simulink model "WDS"  (R2022a)
settings: Solver=FixedStepDiscrete  StartTime=0.0  StopTime=T_final  FixedStep=T_sample  RelTol=1e-3
values from neighbouring files (symbols this model uses):
  A_bar_d = readmatrix('A_bar_d.csv')    [Run_model_WDS.m]
  B_bar_d = readmatrix('B_bar_d.csv')    [Run_model_WDS.m]
  BDD_thresh = 5    [Run_model_WDS.m]    (also in run_model.m = 0.05)
  C_obsv_d = readmatrix('C_obsv_d.csv')    [Run_model_WDS.m]    (also in run_model.m = C_obsv; run_model_power_system.m = C_obsv)
  Cm = ones(1,n_states)    [Run_model_WDS.m]
  D_obsv_d = readmatrix('D_obsv_d.csv')    [Run_model_WDS.m]    (also in run_model.m = D_obsv; run_model_power_system.m = D_obsv)
  eta = 0.7    [Run_model_WDS.m]
  H0_perp_full = eye(size(H0_full,1)) - H0_full*H0_full_pinv    [Run_model_WDS.m]    (also in run_model_power_system.m)
  K = place(A_bar_d,B_bar_d,Pc)    [Run_model_WDS.m]
  k0 = 42    [Run_model_WDS.m]
  Lu = F-A_bar_d.'*H0_full_pinv*H1_full    [Run_model_WDS.m]    (also in run_model_power_system.m)
  Ly = A_bar_d.'*H0_full_pinv    [Run_model_WDS.m]    (also in run_model_power_system.m)
  max_attack = 1000    [Run_model_WDS.m]
  n_attack = round(attack_percentage*n_meas)    [Run_model_WDS.m]    (also in run_model.m = round(0.2*n_meas))
  n_meas = size(C_obsv_d,1)    [Run_model_WDS.m]    (also in run_model.m = n_gen + n_bus; run_model_power_system.m = n_gen + n_bus)
  offset = -inv(B_bar_d)*(A_bar_d-eye(n_states))*xd    [Run_model_WDS.m]
  P = [0.69950062422 0.693508114856 0.716853932584 0.638077403246 0.655805243446 0.637952559301 0.64506866417 0.648938826467 0.678776529338 0.684394506866 0.732584269663 0.692634207241 ... (61 elements, 1x61)]    [P.mat]    (also in Run_model_WDS.m = load('P.mat').P.'; detector_evaluation.m = sum(q==q_hat,1)/(size(q,1)); run_model.m = .1 + .4*rand(2*n_gen,1); run_model_power_system.m = .1 + .4*rand(2*n_gen,1))
  Q0 = ones(n_meas,T)    [Run_model_WDS.m]
  r_tau = chi2inv(0.1,n_meas)    [Run_model_WDS.m]
  Sigma = diag(sigma)    [Run_model_WDS.m]    (also in run_model.m)
  sigma_inv_k = 1e2*(3 + 2*rand(n_meas,1))    [Run_model_WDS.m]    (also in run_model.m = 1e4*(3 + 2*rand(m,1)); sigma_inv_k.mat = [541957.05841 17086.3156535 20847.4062112 958.936090052 8825)
  T = round(2*n_states)    [Run_model_WDS.m]    (also in run_model.m = round(2*n); run_model_power_system.m = 10)
  T_sample = 0.01    [Run_model_WDS.m]    (also in run_model.m; run_model_power_system.m)
  T_start_attack = 0.1*T_final    (= 0.8)    [Run_model_WDS.m]    (also in run_model.m = 1.6; run_model_power_system.m)
  T_start_detect = T_start_attack+T*T_sample    [Run_model_WDS.m]    (also in run_model_power_system.m = 0.9)
  U0 = zeros(n_int,T+1)    [Run_model_WDS.m]    (also in run_model.m = zeros(m,T); run_model_power_system.m)
  x0 = zeros(n_states,1)    [Run_model_WDS.m]    (also in run_model.m; run_model_power_system.m)
  xd = 5*ones(n_states,1)    [Run_model_WDS.m]
  Y0 = zeros(n_meas,T)    [Run_model_WDS.m]    (also in run_model.m = zeros(m,T); run_model_power_system.m)
undefined symbols (not defined in the file or in its folder): F, H0_full, H1_full, T_start_opt
libraries: simulink x10
settings Model: Creator=Abelb  LastModifiedBy=Abelb

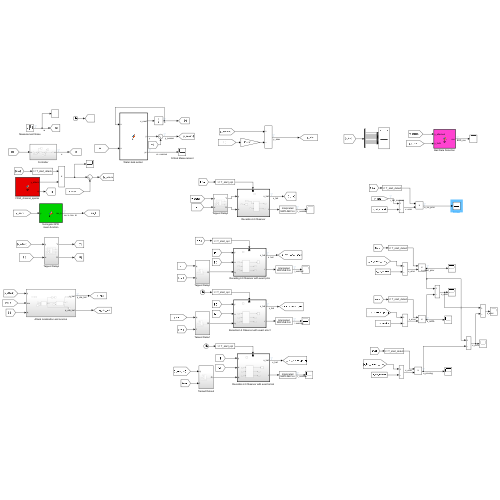
[thumbnail: Simulink's stored preview of the top-level diagram]
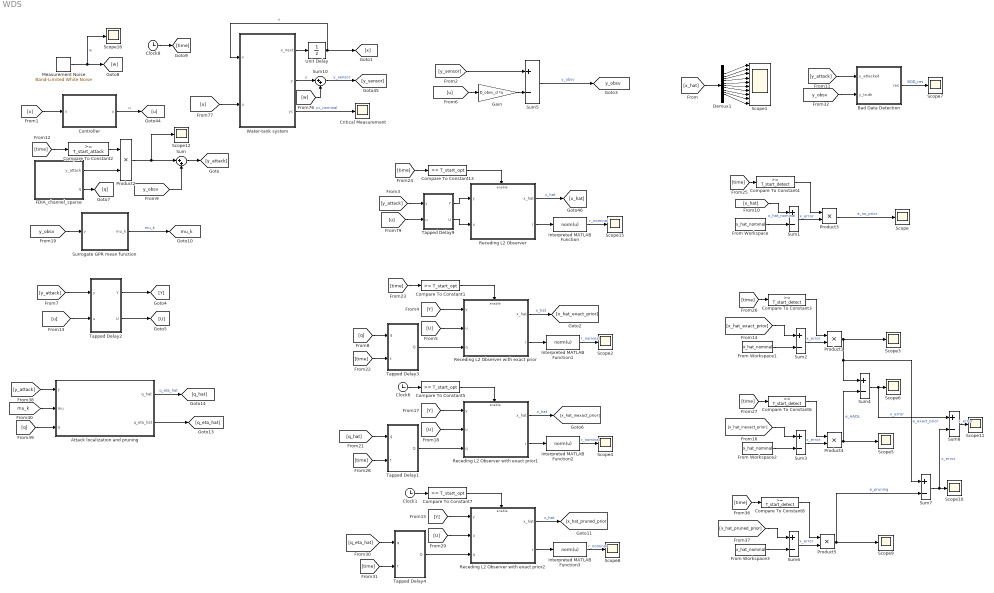
== system WDS ==
  Attack localization and pruning : Subsystem
  Bad Data Detection : MATLAB Function  TreatAsAtomicUnit=on
  Clock1 : Clock
  Clock6 : Clock
  Clock8 : Clock
  Compare To Constant{1,5,7,13} (4 alike) : simulink/Logic and Bit Operations/Compare To Constant  relop=>=  const=T_start_opt  OutDataTypeStr=boolean
  Compare To Constant2 : simulink/Logic and Bit Operations/Compare To Constant  relop=>=  const=T_start_attack  OutDataTypeStr=boolean
  Compare To Constant{3..4,6,8} (4 alike) : simulink/Logic and Bit Operations/Compare To Constant  relop=>=  const=T_start_detect  OutDataTypeStr=boolean
  Controller : Subsystem
  Critical Measurement : Scope
  Demux1 : Demux  Outputs=n_states
  FDIA_channel_sparse : MATLAB Function  TreatAsAtomicUnit=on
  From Workspace{,1..3} (4 alike) : FromWorkspace  VariableName=x_hat_nominal
  Gain : Gain  Gain=D_obsv_d  Multiplication=Matrix(K*u) (u vector)
  Interpreted MATLAB Function{,1..3} (4 alike) : MATLABFcn  MATLABFcn=norm(u)
  Measurement Noise : simulink/Sources/Band-Limited White Noise  Cov=[1e-7]  Ts=T_sample  seed=[23341]
  Product{1..5} (5 alike) : Product
  Receding L2 Observer : Subsystem
  Receding L2 Observer with exact prior : Subsystem
  Receding L2 Observer with exact prior1 : Subsystem
  Receding L2 Observer with exact prior2 : Subsystem
  Scope{,2..12,15..16} (14 alike) : Scope
  Scope1 : Scope  NumInputPorts=10
  Sum : Sum  Inputs=|++
  Sum{1..8} (8 alike) : Sum  Inputs=+-
  Sum10 : Sum  Inputs=|++
  Surrogate GPR mean function : MATLAB Function  TreatAsAtomicUnit=on
  Tapped Delay1 : Subsystem
  Tapped Delay2 : Subsystem
  Tapped Delay3 : Subsystem
  Tapped Delay4 : Subsystem
  Tapped Delay9 : Subsystem
  Unit Delay : UnitDelay  InitialCondition=x0  SampleTime=-1  HasFrameUpgradeWarning=on
  Water-tank system : MATLAB Function  TreatAsAtomicUnit=on
  tag scope: mu_k=global, y_obsv=global
  wires:
  [y_attack] -> Tapped Delay9/1(y)
  Measurement Noise/1 -> Scope16/1, [w]  "w"
  Receding L2 Observer/2(r) -> Interpreted MATLAB Function/1
  Unit Delay/1 -> Water-tank system/1(x), [x]  "x"
  Water-tank system/3(yc) -> Critical Measurement/1  "yc_nominal"
  Interpreted MATLAB Function/1 -> Scope15/1  "r_nominal"
  [w] -> Sum10/2
  [x] -> Controller/1(x)
  Compare To Constant13/1 -> Receding L2 Observer/Enable
  [time] -> Compare To Constant13/1
  Receding L2 Observer/1(x_hat) -> [x_hat]  "x_hat"
  [u] -> Water-tank system/2(u)
  Sum10/1 -> [y_sensor]  "y_sensor"
  Tapped Delay9/1(Y) -> Receding L2 Observer/1(y)
  Controller/1(u) -> [u]  "u"
  Tapped Delay9/2(U) -> Receding L2 Observer/2(u)
  Water-tank system/2(y) -> Sum10/1  "y"
  [u] -> Tapped Delay9/2(u)
  Water-tank system/1(x_next) -> Unit Delay/1
  [y_sensor] -> Sum5/1
  [u] -> Gain/1
  Gain/1 -> Sum5/2
  Sum5/1 -> [y_obsv]  "y_obsv"
  Demux1/1 -> Scope1/1
  Demux1/3 -> Scope1/3
  Demux1/9 -> Scope1/9
  Demux1/6 -> Scope1/6
  Demux1/5 -> Scope1/5
  Demux1/4 -> Scope1/4
  Demux1/8 -> Scope1/8
  Demux1/2 -> Scope1/2
  Demux1/7 -> Scope1/7
  Demux1/10 -> Scope1/10
  [x_hat] -> Demux1/1
  FDIA_channel_sparse/1(y_attack) -> Product2/2
  FDIA_channel_sparse/2(q) -> [q]
  [time] -> Compare To Constant2/1
  Compare To Constant2/1 -> Product2/1
  Product2/1 -> Scope12/1, Sum/1
  [U] -> Receding L2 Observer with exact prior/2(u)
  [Y] -> Receding L2 Observer with exact prior/1(y)
  Receding L2 Observer with exact prior/1(x_hat) -> [x_hat_exact_prior]  "x_hat"
  Compare To Constant1/1 -> Receding L2 Observer with exact prior/Enable
  Interpreted MATLAB Function1/1 -> Scope2/1  "r_nominal"
  Receding L2 Observer with exact prior/2(r) -> Interpreted MATLAB Function1/1
  [time] -> Compare To Constant1/1
  [y_attack] -> Tapped Delay2/1(y)
  Tapped Delay2/2(U) -> [U]
  [time] -> Tapped Delay3/2(t)
  Tapped Delay2/1(Y) -> [Y]
  [q] -> Tapped Delay3/1(q)
  [u] -> Tapped Delay2/2(u)
  [y_obsv] -> Sum/2
  Sum/1 -> [y_attack]
  [x_hat] -> Sum1/1  "x_hat_nominal"
  From Workspace/1 -> Sum1/2
  [y_obsv] -> Bad Data Detection/2(y_truth)
  [y_attack] -> Bad Data Detection/1(y_attacked)
  Bad Data Detection/1(res) -> Scope7/1  "BDD_res"
  Tapped Delay3/1(Q) -> Receding L2 Observer with exact prior/3(q)
  From Workspace1/1 -> Sum2/2
  [x_hat_exact_prior] -> Sum2/1
  Product1/1 -> Sum7/1, Sum4/1, Scope3/1  "e_exact_prior"
  Sum2/1 -> Product1/2  "x_error"
  [time] -> Compare To Constant3/1
  Compare To Constant3/1 -> Product1/1
  [time] -> Compare To Constant4/1
  Compare To Constant4/1 -> Product3/1
  Product3/1 -> Scope/1  "e_no_prior"
  Sum1/1 -> Product3/2  "x_error"
  [time] -> Compare To Constant6/1
  Product4/1 -> Sum4/2, Scope5/1  "e_AADL"
  Compare To Constant6/1 -> Product4/1
  [Y] -> Receding L2 Observer with exact prior1/1(y)
  Clock6/1 -> Compare To Constant5/1
  Compare To Constant5/1 -> Receding L2 Observer with exact prior1/Enable
  From Workspace2/1 -> Sum3/2
  Receding L2 Observer with exact prior1/1(x_hat) -> [x_hat_inexact_prior]  "x_hat"
  [x_hat_inexact_prior] -> Sum3/1
  Interpreted MATLAB Function2/1 -> Scope4/1  "r_nominal"
  Receding L2 Observer with exact prior1/2(r) -> Interpreted MATLAB Function2/1
  Sum3/1 -> Product4/2  "x_error"
  Tapped Delay1/1(Q) -> Receding L2 Observer with exact prior1/3(q)
  [U] -> Receding L2 Observer with exact prior1/2(u)
  [y_obsv] -> Surrogate GPR mean function/1(y)
  Surrogate GPR mean function/1(mu_k) -> [mu_k]  "mu_k"
  Clock8/1 -> [time]
  [q_hat] -> Tapped Delay1/1(q)
  [time] -> Tapped Delay1/2(t)
  Sum4/1 -> Sum8/1, Scope6/1  "x_error"
  Tapped Delay4/1(Q) -> Receding L2 Observer with exact prior2/3(q)
  [time] -> Tapped Delay4/2(t)
  [q_eta_hat] -> Tapped Delay4/1(q)
  Clock1/1 -> Compare To Constant7/1
  [U] -> Receding L2 Observer with exact prior2/2(u)
  Interpreted MATLAB Function3/1 -> Scope8/1  "r_nominal"
  Receding L2 Observer with exact prior2/1(x_hat) -> [x_hat_pruned_prior]  "x_hat"
  Compare To Constant7/1 -> Receding L2 Observer with exact prior2/Enable
  Receding L2 Observer with exact prior2/2(r) -> Interpreted MATLAB Function3/1
  [Y] -> Receding L2 Observer with exact prior2/1(y)
  Product5/1 -> Sum7/2, Scope9/1  "e_pruning"
  Sum6/1 -> Product5/2  "x_error"
  From Workspace3/1 -> Sum6/2
  [time] -> Compare To Constant8/1
  [x_hat_pruned_prior] -> Sum6/1
  Compare To Constant8/1 -> Product5/1
  Sum7/1 -> Sum8/2, Scope10/1  "x_error"
  [mu_k] -> Attack localization and pruning/2(mu)
  [y_attack] -> Attack localization and pruning/1(y)
  [q] -> Attack localization and pruning/3(q)
  Attack localization and pruning/2(q_eta_hat) -> [q_eta_hat]
  Attack localization and pruning/1(q_hat) -> [q_hat]  "q_eta_hat"
  Sum8/1 -> Scope11/1  "x_error"

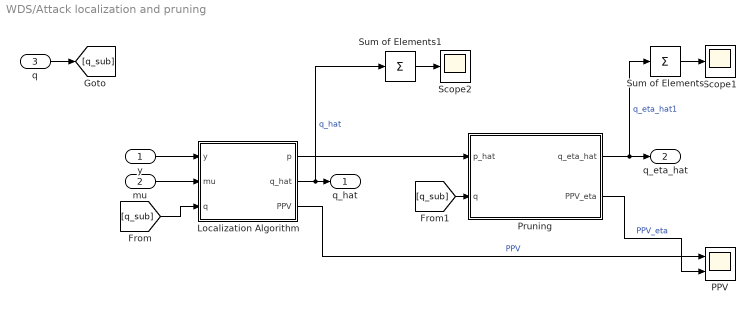
== system WDS/Attack localization and pruning ==
  y : Inport
  mu : Inport  Port=2
  q : Inport  Port=3
  Localization Algorithm : MATLAB Function  TreatAsAtomicUnit=on
  PPV : Scope  NumInputPorts=2
  Pruning : MATLAB Function  TreatAsAtomicUnit=on
  Scope1 : Scope
  Scope2 : Scope
  Sum of Elements : Sum  Inputs=+
  Sum of Elements1 : Sum  Inputs=+
  q_hat : Outport
  q_eta_hat : Outport  Port=2
  wires:
  y/1 -> Localization Algorithm/1(y)
  mu/1 -> Localization Algorithm/2(mu)
  Localization Algorithm/3(PPV) -> PPV/1  "PPV"
  Localization Algorithm/2(q_hat) -> Sum of Elements1/1, q_hat/1  "q_hat"
  Localization Algorithm/1(p) -> Pruning/1(p_hat)
  Pruning/2(PPV_eta) -> PPV/2  "PPV_eta"
  q/1 -> [q_sub]
  [q_sub] -> Localization Algorithm/3(q)
  [q_sub] -> Pruning/2(q)
  Sum of Elements/1 -> Scope1/1
  Pruning/1(q_eta_hat) -> Sum of Elements/1, q_eta_hat/1  "q_eta_hat1"
  Sum of Elements1/1 -> Scope2/1

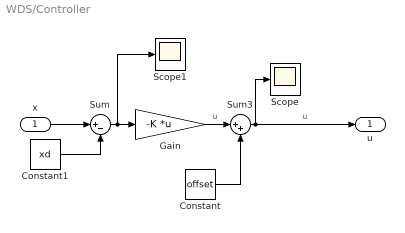
== system WDS/Controller ==
  x : Inport
  Constant : Constant  Value=offset
  Constant1 : Constant  Value=xd
  Gain : Gain  Gain=-K  Multiplication=Matrix(K*u) (u vector)
  Scope : Scope
  Scope1 : Scope
  Sum : Sum  Inputs=|+-
  Sum3 : Sum  Inputs=|++
  u : Outport
  wires:
  Sum3/1 -> u/1, Scope/1  "u"
  Constant/1 -> Sum3/2
  Constant1/1 -> Sum/2
  Gain/1 -> Sum3/1  "u"
  Sum/1 -> Scope1/1, Gain/1
  x/1 -> Sum/1

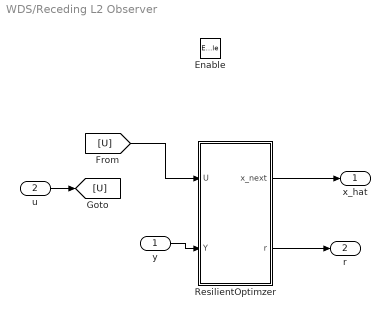
== system WDS/Receding L2 Observer ==
  y : Inport
  u : Inport  Port=2
  Enable : EnablePort
  ResilientOptimzer : MATLAB Function  TreatAsAtomicUnit=on
  x_hat : Outport
  r : Outport  Port=2
  wires:
  u/1 -> [U]
  y/1 -> ResilientOptimzer/2(Y)
  [U] -> ResilientOptimzer/1(U)
  ResilientOptimzer/1(x_next) -> x_hat/1
  ResilientOptimzer/2(r) -> r/1

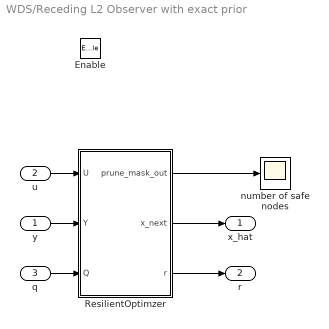
== system WDS/Receding L2 Observer with exact prior ==
  y : Inport
  u : Inport  Port=2
  q : Inport  Port=3
  Enable : EnablePort
  ResilientOptimzer : MATLAB Function  TreatAsAtomicUnit=on
  number of safe nodes : Scope
  x_hat : Outport
  r : Outport  Port=2
  wires:
  y/1 -> ResilientOptimzer/2(Y)
  ResilientOptimzer/2(x_next) -> x_hat/1
  ResilientOptimzer/3(r) -> r/1
  u/1 -> ResilientOptimzer/1(U)
  q/1 -> ResilientOptimzer/3(Q)
  ResilientOptimzer/1(prune_mask_out) -> number of safe nodes/1

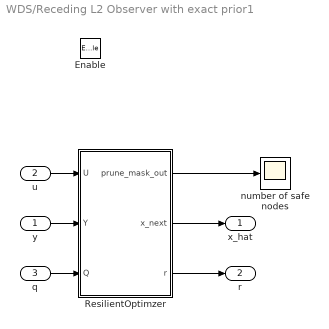
== system WDS/Receding L2 Observer with exact prior1 ==
  y : Inport
  u : Inport  Port=2
  q : Inport  Port=3
  Enable : EnablePort
  ResilientOptimzer : MATLAB Function  TreatAsAtomicUnit=on
  number of safe nodes : Scope
  x_hat : Outport
  r : Outport  Port=2
  wires:
  y/1 -> ResilientOptimzer/2(Y)
  ResilientOptimzer/2(x_next) -> x_hat/1
  ResilientOptimzer/3(r) -> r/1
  u/1 -> ResilientOptimzer/1(U)
  q/1 -> ResilientOptimzer/3(Q)
  ResilientOptimzer/1(prune_mask_out) -> number of safe nodes/1

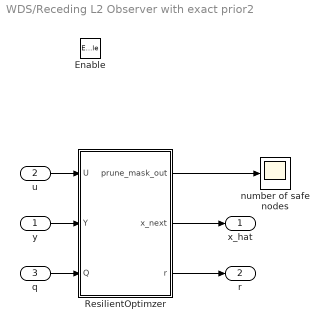
== system WDS/Receding L2 Observer with exact prior2 ==
  y : Inport
  u : Inport  Port=2
  q : Inport  Port=3
  Enable : EnablePort
  ResilientOptimzer : MATLAB Function  TreatAsAtomicUnit=on
  number of safe nodes : Scope
  x_hat : Outport
  r : Outport  Port=2
  wires:
  y/1 -> ResilientOptimzer/2(Y)
  ResilientOptimzer/2(x_next) -> x_hat/1
  ResilientOptimzer/3(r) -> r/1
  u/1 -> ResilientOptimzer/1(U)
  q/1 -> ResilientOptimzer/3(Q)
  ResilientOptimzer/1(prune_mask_out) -> number of safe nodes/1

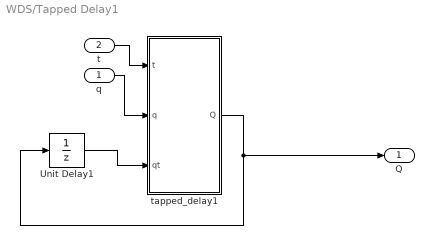
== system WDS/Tapped Delay1 ==
  q : Inport
  t : Inport  Port=2
  Unit Delay1 : UnitDelay  InitialCondition=Q0  SampleTime=-1  HasFrameUpgradeWarning=on
  tapped_delay1 : MATLAB Function  TreatAsAtomicUnit=on
  Q : Outport
  wires:
  t/1 -> tapped_delay1/1(t)
  Unit Delay1/1 -> tapped_delay1/3(qt)
  tapped_delay1/1(Q) -> Q/1, Unit Delay1/1
  q/1 -> tapped_delay1/2(q)

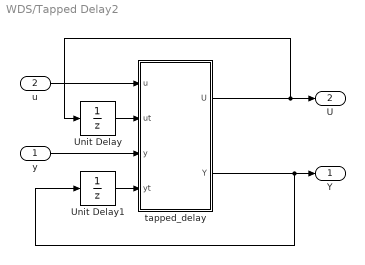
== system WDS/Tapped Delay2 ==
  y : Inport
  u : Inport  Port=2
  Unit Delay : UnitDelay  InitialCondition=U0  SampleTime=-1  HasFrameUpgradeWarning=on
  Unit Delay1 : UnitDelay  InitialCondition=Y0  SampleTime=-1  HasFrameUpgradeWarning=on
  tapped_delay : MATLAB Function  TreatAsAtomicUnit=on
  Y : Outport
  U : Outport  Port=2
  wires:
  u/1 -> tapped_delay/1(u)
  y/1 -> tapped_delay/3(y)
  tapped_delay/1(U) -> Unit Delay/1, U/1
  tapped_delay/2(Y) -> Unit Delay1/1, Y/1
  Unit Delay/1 -> tapped_delay/2(ut)
  Unit Delay1/1 -> tapped_delay/4(yt)

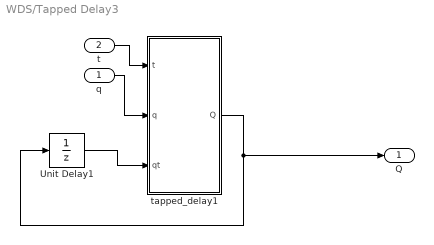
== system WDS/Tapped Delay3 ==
  q : Inport
  t : Inport  Port=2
  Unit Delay1 : UnitDelay  InitialCondition=Q0  SampleTime=-1  HasFrameUpgradeWarning=on
  tapped_delay1 : MATLAB Function  TreatAsAtomicUnit=on
  Q : Outport
  wires:
  t/1 -> tapped_delay1/1(t)
  Unit Delay1/1 -> tapped_delay1/3(qt)
  tapped_delay1/1(Q) -> Q/1, Unit Delay1/1
  q/1 -> tapped_delay1/2(q)

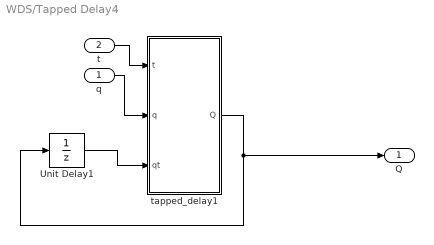
== system WDS/Tapped Delay4 ==
  q : Inport
  t : Inport  Port=2
  Unit Delay1 : UnitDelay  InitialCondition=Q0  SampleTime=-1  HasFrameUpgradeWarning=on
  tapped_delay1 : MATLAB Function  TreatAsAtomicUnit=on
  Q : Outport
  wires:
  t/1 -> tapped_delay1/1(t)
  Unit Delay1/1 -> tapped_delay1/3(qt)
  tapped_delay1/1(Q) -> Q/1, Unit Delay1/1
  q/1 -> tapped_delay1/2(q)

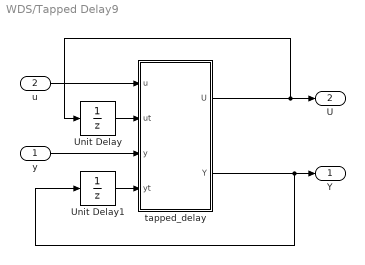
== system WDS/Tapped Delay9 ==
  y : Inport
  u : Inport  Port=2
  Unit Delay : UnitDelay  InitialCondition=U0  SampleTime=-1  HasFrameUpgradeWarning=on
  Unit Delay1 : UnitDelay  InitialCondition=Y0  SampleTime=-1  HasFrameUpgradeWarning=on
  tapped_delay : MATLAB Function  TreatAsAtomicUnit=on
  Y : Outport
  U : Outport  Port=2
  wires:
  u/1 -> tapped_delay/1(u)
  y/1 -> tapped_delay/3(y)
  tapped_delay/1(U) -> Unit Delay/1, U/1
  tapped_delay/2(Y) -> Unit Delay1/1, Y/1
  Unit Delay/1 -> tapped_delay/2(ut)
  Unit Delay1/1 -> tapped_delay/4(yt)

== matlab function WDS/Tapped Delay4/tapped_delay1 ==
  data: t input; q input; qt input; Q output; n_meas parameter; T_start_attack parameter; T parameter
function Q  = fcn(t, q,qt,n_meas,T_start_attack, T)
%% tapped_delay_array
% shift columns from tapped matrix to the left and appends most recent
% vector to the last column
% %%% input
% ut(:,1:end-1) = ut(:,2:end);
% ut(:,end) = u;
% U = ut;
% %%% output
% yt(:,1:end-1) = yt(:,2:end);
% yt(:,end) = y;
% Y = yt;
%%% pruning support
Q = ones(n_meas,T);
if t>T_start_attack
    qt(:,1:end-1) = qt(:,2:end);
    qt(:,end) = q;
    Q = qt;
end
end

== matlab function WDS/Tapped Delay3/tapped_delay1 ==
  data: t input; q input; qt input; Q output; n_meas parameter; T_start_attack parameter; T parameter
function Q  = fcn(t, q,qt,n_meas,T_start_attack, T)
%% tapped_delay_array
% shift columns from tapped matrix to the left and appends most recent
% vector to the last column
% %%% input
% ut(:,1:end-1) = ut(:,2:end);
% ut(:,end) = u;
% U = ut;
% %%% output
% yt(:,1:end-1) = yt(:,2:end);
% yt(:,end) = y;
% Y = yt;
%%% pruning support
Q = ones(n_meas,T);
if t>T_start_attack
    qt(:,1:end-1) = qt(:,2:end);
    qt(:,end) = q;
    Q = qt;
end
end

== matlab function WDS/Receding L2 Observer/ResilientOptimzer ==
  data: x_next output; U input; Y input; Ly parameter; Lu parameter; H0_perp_full parameter; H1_full parameter; r output
function [x_next,r]  = fcn(U,Y, Ly, Lu,H0_perp_full, H1_full)


u_local = U(:,1:end-1);
% vectorized
u = u_local(:);
y = Y(:);

x_next = zeros(10,1);
x_next(:) = Ly*y + Lu*u;

r = H0_perp_full*(y-H1_full*u);

== matlab function WDS/FDIA_channel_sparse ==
  data: n_attack parameter; y_attack output; n_meas parameter; C_obsv_d parameter; max_attack parameter; BDD_thresh parameter; q output
function [y_attack,q] = fcn(n_attack,n_meas,C_obsv_d,max_attack, BDD_thresh)

%% Measurement Channel Attack
%  Assumptions:
%  1. The attacker knows the actual measurement
%  2. The attacker can only corrupt upto n_attack measurements
%  3. The attacker knows the BDD theshold

attack_idx = randi(n_meas,n_attack,1);
% attack_idx = [10; 18];
y_attack   = gen_attack_channel(C_obsv_d, max_attack,attack_idx,BDD_thresh);
                                                        % NOTE THE .75
                                                        % Used
                                                        % conservatively
q = ones(n_meas,1);
q(attack_idx) = 0;

== matlab function WDS/Bad Data Detection ==
  data: y_attacked input; y_truth input; res output; U2 parameter
function res = fcn(y_attacked,y_truth,U2)

res = [norm(U2.'*y_attacked,2);
       norm(U2.'*y_truth,2)];

== matlab function WDS/Attack localization and pruning/Localization Algorithm ==
  data: p output; y input; q_hat output; mu input; Sigma parameter; n_meas parameter; q input; PPV output
function [p, q_hat,PPV] = fcn(y,mu,Sigma, n_meas,q)

%% calculate probability
z = (y - mu)./diag(Sigma);
p = 2*(ones(n_meas,1)-normcdf(abs(z)));

%% support prior and corresponding confidence
% q_hat = zeros(n_meas,1);
% q_hat(p <= 0.5) = 1;
q_hat = double(p>=0.5);

PPV = sum(q.*q_hat)/sum(q_hat);

== matlab function WDS/Attack localization and pruning/Pruning ==
  data: p_hat input; q_eta_hat output; eta parameter; n_meas parameter; PPV_eta output; k0 parameter; q input; P parameter
function [q_eta_hat,PPV_eta] = fcn(p_hat,eta, n_meas,k0, q, P)

q_eta_hat = ones(n_meas,1);
coder.extrinsic('pruning_algorithm2')
q_eta_hat = pruning_algorithm2(p_hat,P,eta,k0);


PPV_eta = sum(q.*q_eta_hat)/sum(q_eta_hat);
end

== matlab function WDS/Tapped Delay9/tapped_delay ==
  data: u input; U output; ut input; y input; yt input; Y output
function [U,Y] = fcn(u,ut,y,yt)
%% tapped_delay_array
% shift columns from tapped matrix to the left and appends most recent
% vector to the last column
%%% input
ut(:,1:end-1) = ut(:,2:end);
ut(:,end) = u;
U = ut;
%%% output
yt(:,1:end-1) = yt(:,2:end);
yt(:,end) = y;
Y = yt;

== matlab function WDS/Water-tank system ==
  data: x input; x_next output; u input; y output; A_bar_d parameter; C_obsv_d parameter; B_bar_d parameter; D_obsv_d parameter; yc output; Cm parameter
function [x_next,y,yc] = fcn(x,u,A_bar_d,C_obsv_d,B_bar_d,D_obsv_d,Cm)
% Discrete state-space model for system

x_next = A_bar_d*x + B_bar_d*u ;

y = C_obsv_d*x + D_obsv_d*u;

% critical measurements
yc = Cm*x;

== matlab function WDS/Receding L2 Observer with exact prior/ResilientOptimzer ==
  data: prune_mask_out output; x_next output; U input; Y input; H0_perp_full parameter; H0_full parameter; H1_full parameter; r output; Q input; F parameter; A_bar_d parameter
function [prune_mask_out, x_next,r]  = fcn(U,Y,H0_perp_full, H0_full, H1_full, Q, F, A_bar_d)


u_local = U(:,1:end-1);
% vectorized
u = u_local(:);
y = Y(:);
q = Q(:);

n_states = size(A_bar_d,1);

%% pruning
prune_mask_out = sum(q>0.5);   % mask for safe nodes
prune_mask = find(q>0.5); %find(q_eta_hat>0.5); % true(size(q_eta_hat,1),1);

H0_eta = H0_full(prune_mask,:);
H1_eta = H1_full(prune_mask,:);

H0_eta_pinv = pinv(H0_eta,0.001);
Ly = A_bar_d.'*H0_eta_pinv;
Lu = F-A_bar_d.'*H0_eta_pinv*H1_eta;

x_next = zeros(n_states,1);
x_next(:) = Ly*y(prune_mask) + Lu*u;

r = H0_perp_full*(y-H1_full*u);

== matlab function WDS/Receding L2 Observer with exact prior1/ResilientOptimzer ==
  data: prune_mask_out output; x_next output; U input; Y input; H0_perp_full parameter; H0_full parameter; H1_full parameter; r output; Q input; F parameter; A_bar_d parameter
function [prune_mask_out, x_next,r]  = fcn(U,Y,H0_perp_full, H0_full, H1_full, Q, F, A_bar_d)


u_local = U(:,1:end-1);
% vectorized
u = u_local(:);
y = Y(:);
q = Q(:);

n_states = size(A_bar_d,1);

%% pruning
prune_mask_out = sum(q>0.5);   % mask for safe nodes
prune_mask = find(q>0.5); %find(q_eta_hat>0.5); % true(size(q_eta_hat,1),1);

H0_eta = H0_full(prune_mask,:);
H1_eta = H1_full(prune_mask,:);

H0_eta_pinv = pinv(H0_eta,0.001);
Ly = A_bar_d.'*H0_eta_pinv;
Lu = F-A_bar_d.'*H0_eta_pinv*H1_eta;

x_next = zeros(n_states,1);
x_next(:) = Ly*y(prune_mask) + Lu*u;

r = H0_perp_full*(y-H1_full*u);

== matlab function WDS/Tapped Delay2/tapped_delay ==
  data: u input; U output; ut input; y input; yt input; Y output
function [U,Y] = fcn(u,ut,y,yt)
%% tapped_delay_array
% shift columns from tapped matrix to the left and appends most recent
% vector to the last column
%%% input
ut(:,1:end-1) = ut(:,2:end);
ut(:,end) = u;
U = ut;
%%% output
yt(:,1:end-1) = yt(:,2:end);
yt(:,end) = y;
Y = yt;

== matlab function WDS/Tapped Delay1/tapped_delay1 ==
  data: t input; q input; qt input; Q output; n_meas parameter; T_start_attack parameter; T parameter
function Q  = fcn(t, q,qt,n_meas,T_start_attack, T)
%% tapped_delay_array
% shift columns from tapped matrix to the left and appends most recent
% vector to the last column
% %%% input
% ut(:,1:end-1) = ut(:,2:end);
% ut(:,end) = u;
% U = ut;
% %%% output
% yt(:,1:end-1) = yt(:,2:end);
% yt(:,end) = y;
% Y = yt;
%%% pruning support
Q = ones(n_meas,T);
if t>T_start_attack
    qt(:,1:end-1) = qt(:,2:end);
    qt(:,end) = q;
    Q = qt;
end
end

== matlab function WDS/Surrogate GPR mean function ==
  data: y input; mu_k output; sigma_inv_k parameter; r_tau parameter; n_meas parameter
function mu_k = fcn(y,sigma_inv_k, r_tau,n_meas)
% Prunes a random vector to find mu_k so that ||y-mu_k||_Sigma_inv_k <= r_tau

% first: random vector, secomd: normalize
y_rand = rand(n_meas,1);
y_rand = sqrt(r_tau/max(sigma_inv_k))/norm(y_rand)*y_rand;

% create mu_k from y
mu_k = y - y_rand;

% mu_k = (U_y_1*U_y_1.')*y;

== matlab function WDS/Receding L2 Observer with exact prior2/ResilientOptimzer ==
  data: prune_mask_out output; x_next output; U input; Y input; H0_perp_full parameter; H0_full parameter; H1_full parameter; r output; Q input; F parameter; A_bar_d parameter
function [prune_mask_out, x_next,r]  = fcn(U,Y,H0_perp_full, H0_full, H1_full, Q, F, A_bar_d)


u_local = U(:,1:end-1);
% vectorized
u = u_local(:);
y = Y(:);
q = Q(:);

n_states = size(A_bar_d,1);

%% pruning
prune_mask_out = sum(q>0.5);   % mask for safe nodes
prune_mask = find(q>0.5); %find(q_eta_hat>0.5); % true(size(q_eta_hat,1),1);

H0_eta = H0_full(prune_mask,:);
H1_eta = H1_full(prune_mask,:);

H0_eta_pinv = pinv(H0_eta,0.001);
Ly = A_bar_d.'*H0_eta_pinv;
Lu = F-A_bar_d.'*H0_eta_pinv*H1_eta;

x_next = zeros(n_states,1);
x_next(:) = Ly*y(prune_mask) + Lu*u;

r = H0_perp_full*(y-H1_full*u);
